simulink model "Q1_2_1"  (R2020b)
settings: Solver=VariableStepAuto  StartTime=0.0  StopTime=100.0  RelTol=1e-3
settings Model: Creator=kushagrakhatwani  LastModifiedBy=kushagrakhatwani

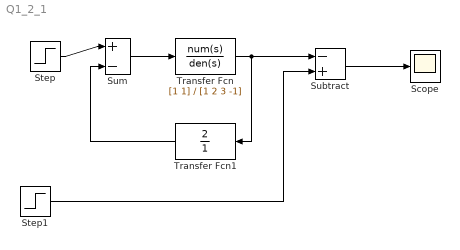
== system Q1_2_1 ==
  Scope : Scope
  Step : Step  Time=0  SampleTime=0
  Step1 : Step  Time=0  SampleTime=0
  Subtract : Sum  Inputs=-+
  Sum : Sum  Inputs=|+-
  Transfer Fcn : TransferFcn  Numerator=[1 1]  Denominator=[1 2 3 -1]
  Transfer Fcn1 : TransferFcn  Numerator=[2]  Denominator=[1]
  wires:
  Transfer Fcn1/1 -> Sum/2
  Step/1 -> Sum/1
  Sum/1 -> Transfer Fcn/1
  Subtract/1 -> Scope/1
  Transfer Fcn/1 -> Transfer Fcn1/1, Subtract/1
  Step1/1 -> Subtract/2
